simulink model "analog_adder"  (R2020b)
settings: Solver=VariableStepAuto  StartTime=0.0  StopTime=10.0  RelTol=1e-3  AbsTol=1e-3
libraries: analogCompBlocks x4, ee_lib x2, fl_lib x1, nesl_utility x1
settings Model: DataDictionary=analogComputerData.sldd  EnableAccessToBaseWorkspace=off  Creator=roadrunner  LastModifiedBy=roadrunner
settings SolverCC: AutoScaleAbsTol=off
settings DebuggingCC: SymbolicDimsDataTypeCodeGenerationDiagnostic=none
settings SFSimCC: CustomCodeUndefinedFunction=UseInterfaceOnly
settings SimscapeCC: SimscapeLogType=all  SimscapeLogSimulationStatistics=on  SimscapeLogDataHistory=10000

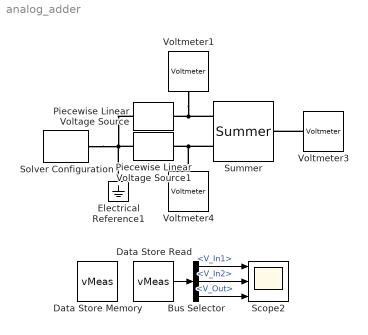
== system analog_adder ==
  Bus Selector : BusSelector  OutputSignals=V_In1,V_In2,V_Out
  Data Store Memory : DataStoreMemory  DataStoreName=vMeas  ReadBeforeWriteMsg=warning  WriteAfterWriteMsg=warning  WriteAfterReadMsg=warning  ShowAdditionalParam=off  OutDataTypeStr=Bus: bus_summer_measurements
  Data Store Read : DataStoreRead  DataStoreName=vMeas
  Electrical Reference1 : fl_lib/Electrical/Electrical Elements/Electrical Reference
  Piecewise Linear Voltage Source : ee_lib/Additional Components/SPICE Sources/Piecewise Linear Voltage Source  TIMElist=[0 2 2.01 6 6.01 10] s  VOLTlist=[0 0 5 5 -5 -5]/2 V  INTERP=1  EXTRAP=2
      settings: SourceProductBaseCode=PS  InternalSimscapePortConfiguration="{\"Bottom\":[],\"Left\":[{\"id\":\"p\",\"label\":\"+\",\"type\":\"foundation.electrical.electrical\"}],\"Right\":[{\"id\":\"n\",\"label\":\"-\",\"type\":\"foundation.electrical.electrical\"}],\"Top\":[]}"
  Piecewise Linear Voltage Source1 : ee_lib/Additional Components/SPICE Sources/Piecewise Linear Voltage Source  TIMElist=[0 2 2.01 6 6.01 10] s  VOLTlist=[0 0 5 5 -5 -5] V  INTERP=1  EXTRAP=2
      settings: SourceProductBaseCode=PS  InternalSimscapePortConfiguration="{\"Bottom\":[],\"Left\":[{\"id\":\"p\",\"label\":\"+\",\"type\":\"foundation.electrical.electrical\"}],\"Right\":[{\"id\":\"n\",\"label\":\"-\",\"type\":\"foundation.electrical.electrical\"}],\"Top\":[]}"
  Scope2 : Scope  NumInputPorts=3
  Solver Configuration : nesl_utility/Solver Configuration  PhysicalDomain=network_engine_domain  SubClassName=solver  LeftPortType=input  RightPortType=generic  Tones=[]  Harmonics=[]  SimulateNoise=off  Profile=off  UseLocalSampling=off  EnableSwitchedLinearOptims=on  FrequencyDomain=off  UseCCode=off  RelTol=0.001  AbsTol=1e-06  MinStep=1e-09  ToWorkspace=off  RevertToSquareIcSolve=off  NumHomotopyIterations=100  PhasorMode=off  PhasorModeNumHarmonics=1  DoDC=off  ResidualTolerance=1e-09  UseLocalSolver=on  LocalSolverChoice=NE_BACKWARD_EULER_ADVANCER  LocalSolverSampleTime=0.01  DoFixedCost=on  MaxNonlinIter=3  MaxModeIter=2  ComputeImpulses=off  ImpulseIterations=2  LinearAlgebra=auto  EquationFormulation=NE_TIME_EF  DelaysMemoryBudget=1024  AutomaticFiltering=on  FilteringTimeConstant=0.001  PartitionStorageMethod=AS_NEEDED  PartitionMemoryBudget=1024  PartitionMethod=ROBUST
      settings: SourceProductName=Utilities
  Summer : analogCompBlocks/Summer  SystemSampleTime=-1  VariantActivationTime=update diagram  Latency=0  AutoFrameSizeCalculation=off
      settings: AttributesFormatString=Summer
  Voltmeter1 : analogCompBlocks/Voltmeter  DSNAME='vMeas'  DSELEMENT='V_In1'
      settings: AttributesFormatString=Voltage Sensor
  Voltmeter3 : analogCompBlocks/Voltmeter  DSNAME='vMeas'  DSELEMENT='V_Out'
      settings: AttributesFormatString=Voltage Sensor
  Voltmeter4 : analogCompBlocks/Voltmeter  DSNAME='vMeas'  DSELEMENT='V_In2'
      settings: AttributesFormatString=Voltage Sensor
  wires:
  Bus Selector/2 -> Scope2/2  "<V_In2>"
  Data Store Read/1 -> Bus Selector/1
  Bus Selector/1 -> Scope2/1  "<V_In1>"
  Bus Selector/3 -> Scope2/3  "<V_Out>"
  connections:
  Electrical Reference1/LConn1 -- Piecewise Linear Voltage Source1/RConn1 -- Piecewise Linear Voltage Source/RConn1 -- Solver Configuration/RConn1
  Summer/LConn1 -- Voltmeter1/LConn1 -- Piecewise Linear Voltage Source/LConn1
  Summer/LConn2 -- Voltmeter4/LConn1 -- Piecewise Linear Voltage Source1/LConn1
  Voltmeter3/LConn1 -- Summer/RConn1
